simulink model "tm_kalman_test"  (R2015a)
settings: Solver=ode45  StartTime=0.0  StopTime=10.0  RelTol=1e-3
undefined symbols (not defined in the file): A, A1, B, B1, beta, C, C1, D, D1, P1, Q1, R1, Ts, x0, x1
libraries: simulink x2, dspsigops x1
settings Model: Creator=Trancemania  LastModifiedBy=Trancemania

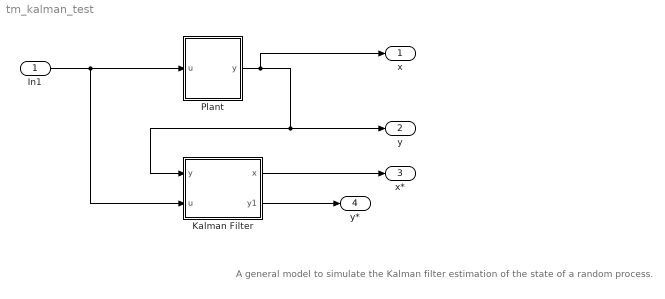
== system tm_kalman_test ==
  note: A general model to simulate the Kalman filter estimation of the state of a random process.
  In1 : Inport
  Kalman Filter : Subsystem  mask{x0=x1, P0=P1, A=A1, B=B1, C=C1, D=D1, Q=Q1, R=R1}
      mask help:
      | Linear Random Process
      | x(k+1)=Ax(k)+Bu(k)+w
      | y(k)=Cx(k)+Du(k)+v
      | w~N(0,Q)
      | w~N(0,R)
      mask Display:
      | disp(sprintf('Kalman\n Filter'))
      | port_label('output',2,'y')
      | port_label('output',1,'x')
      | port_label('input',1,'y')
      | port_label('input',2,'u')
  Plant : Subsystem
  x : Outport
  y : Outport  Port=2
  x* : Outport  Port=3
  y* : Outport  Port=4
  wires:
  In1/1 -> Plant/1(u), Kalman Filter/2(u)
  Plant/1(y) -> x/1, Kalman Filter/1(y), y/1
  Kalman Filter/1(x) -> x*/1
  Kalman Filter/2(y1) -> y*/1

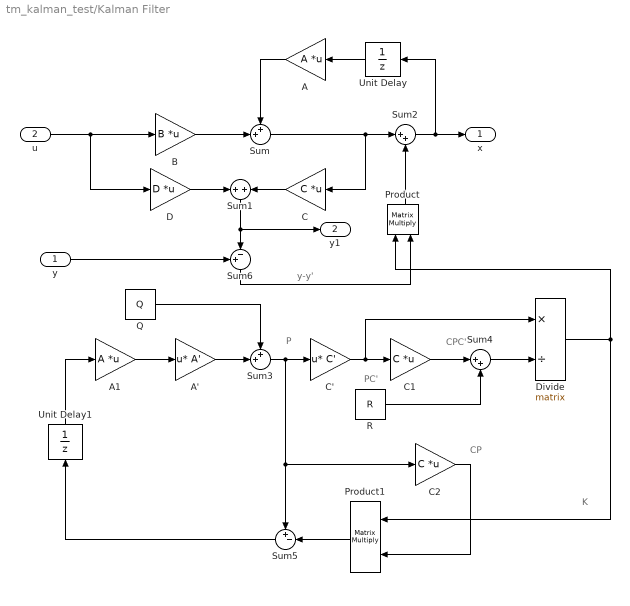
== system tm_kalman_test/Kalman Filter ==
  note: P
  note: PC'
  note: CPC'
  note: K
  note: CP
  note: y-y'
  y : Inport
  u : Inport  Port=2  PortDimensions=size(B,2)
  A : Gain  Gain=A  Multiplication=Matrix(K*u)
  A' : Gain  Gain=A'  Multiplication=Matrix(u*K)
  A1 : Gain  Gain=A  Multiplication=Matrix(K*u)
  B : Gain  Gain=B  Multiplication=Matrix(K*u)
  C : Gain  Gain=C  Multiplication=Matrix(K*u)
  C' : Gain  Gain=C'  Multiplication=Matrix(u*K)
  C1 : Gain  Gain=C  Multiplication=Matrix(K*u)
  C2 : Gain  Gain=C  Multiplication=Matrix(K*u)
  D : Gain  Gain=D  Multiplication=Matrix(K*u)
  Divide : Product  Inputs=*/  Multiplication=Matrix(*)
  Product : Product  Multiplication=Matrix(*)  RndMeth=Zero
  Product1 : Product  Multiplication=Matrix(*)  RndMeth=Zero
  Q : Constant  Value=Q
  R : Constant  Value=R
  Sum : Sum  Inputs=++|
  Sum1 : Sum  Inputs=+|+
  Sum2 : Sum  Inputs=|++
  Sum3 : Sum  Inputs=++|
  Sum4 : Sum  Inputs=|++
  Sum5 : Sum  Inputs=+-|
  Sum6 : Sum  Inputs=+-|
  Unit Delay : UnitDelay  InitialCondition=x0
  Unit Delay1 : UnitDelay  InitialCondition=P0
  x : Outport
  y1 : Outport  Port=2
  wires:
  u/1 -> B/1, D/1
  B/1 -> Sum/2
  A/1 -> Sum/1
  Unit Delay/1 -> A/1
  Sum/1 -> Sum2/1, C/1
  Sum2/1 -> x/1, Unit Delay/1
  D/1 -> Sum1/1
  C/1 -> Sum1/2
  A1/1 -> A'/1
  A'/1 -> Sum3/2
  Q/1 -> Sum3/1
  Sum3/1 -> C'/1, Sum5/1, C2/1
  C'/1 -> C1/1, Divide/1
  Product/1 -> Sum2/2
  Divide/1 -> Product/1, Product1/1
  Product1/1 -> Sum5/2
  C1/1 -> Sum4/1
  R/1 -> Sum4/2
  Sum4/1 -> Divide/2
  Unit Delay1/1 -> A1/1
  Sum5/1 -> Unit Delay1/1
  C2/1 -> Product1/2
  Sum1/1 -> Sum6/2, y1/1
  y/1 -> Sum6/1
  Sum6/1 -> Product/2

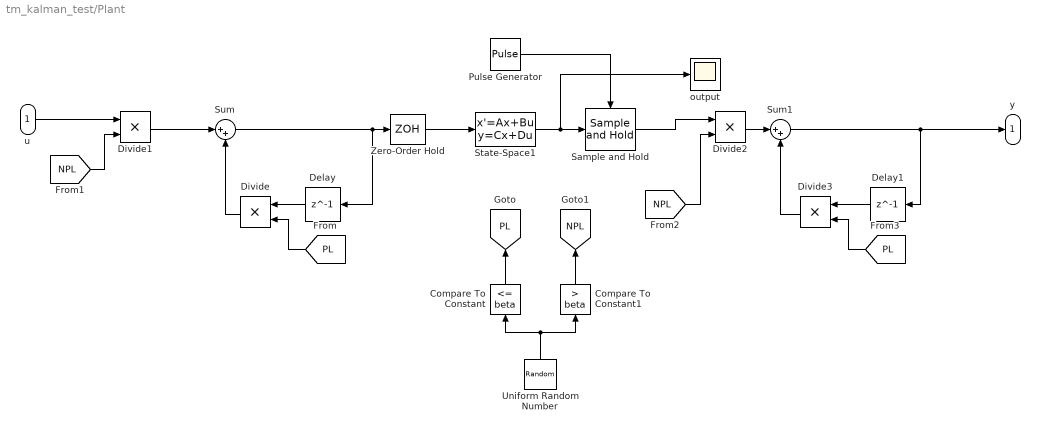
== system tm_kalman_test/Plant ==
  u : Inport
  Compare To Constant : simulink/Logic and Bit Operations/Compare To Constant  relop=<=  const=beta  OutDataTypeStr=boolean
  Compare To Constant1 : simulink/Logic and Bit Operations/Compare To Constant  relop=>  const=beta  OutDataTypeStr=boolean
  Delay : Delay  DelayLength=1  SampleTime=Ts
  Delay1 : Delay  DelayLength=1  SampleTime=Ts
  Divide : Product  Inputs=**
  Divide1 : Product  Inputs=**  SampleTime=Ts
  Divide2 : Product  Inputs=**  SampleTime=Ts
  Divide3 : Product  Inputs=**  SampleTime=Ts
  Pulse Generator : DiscretePulseGenerator  PulseType=Time based  Period=Ts  PulseWidth=5
  Sample and Hold : dspsigops/Sample and Hold  trig=Rising edge  initCond=0  latchinput=off
  State-Space1 : StateSpace  A=A  B=B  C=C  D=D  X0=x0
  Sum : Sum  Inputs=|++  SampleTime=Ts
  Sum1 : Sum  Inputs=|++  SampleTime=Ts
  Uniform Random Number : UniformRandomNumber  Minimum=0  Seed=randi(1000000)  SampleTime=Ts
  Zero-Order Hold : ZeroOrderHold  SampleTime=Ts
  output : Scope
      settings: SaveName=ScopeData3
  y : Outport
  tag scope: NPL=global, PL=global
  wires:
  u/1 -> Divide1/1
  Sum1/1 -> y/1, Delay1/1
  Zero-Order Hold/1 -> State-Space1/1
  State-Space1/1 -> output/1, Sample and Hold/1
  Divide1/1 -> Sum/1
  Sum/1 -> Delay/1, Zero-Order Hold/1
  Uniform Random Number/1 -> Compare To Constant1/1, Compare To Constant/1
  Compare To Constant/1 -> [PL]
  Compare To Constant1/1 -> [NPL]
  Divide/1 -> Sum/2
  [NPL] -> Divide1/2
  Delay/1 -> Divide/1
  [PL] -> Divide/2
  [NPL] -> Divide2/2
  Divide2/1 -> Sum1/1
  Sample and Hold/1 -> Divide2/1
  Delay1/1 -> Divide3/1
  [PL] -> Divide3/2
  Divide3/1 -> Sum1/2
  Pulse Generator/1 -> Sample and Hold/Trigger
